simulink model "REV2_System_Model"  (R2024a)
settings: Solver=VariableStepAuto  StartTime=0.0  StopTime=10.0  RelTol=1e-3
settings Model: Creator=aniru  LastModifiedBy=aniru

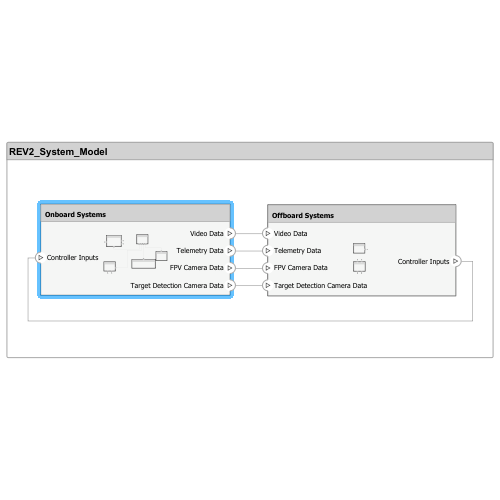
[thumbnail: Simulink's stored preview of the top-level diagram]
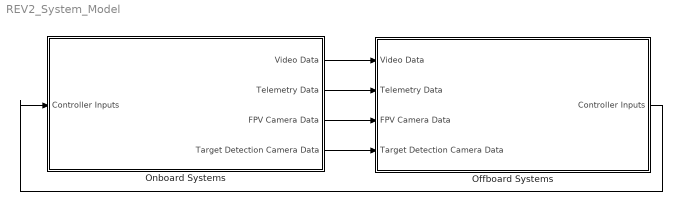
== system REV2_System_Model ==
  Offboard Systems : Subsystem
      settings: PortSchema="{\"entries\":[{\"content\":{\"headerSize\":26,\"margin\":15,\"minimumSpacing\":25,\"sides\":[{\"content\":{\"connectorIds\":[\"In2\",\"In1\",\"In4\",\"In3\"]},\"type\":\"ConnectorPlacement.EquallySpacedRectSide\",\"uuid\":\"d7d6a46a-69a6-4a79-809b-721a0c8eab4f\"},{\"content\":{\"connectorIds\":[\"Out1\"],\"side\":\"RIGHT\"},\"type\":\"ConnectorPlacement.EquallySpacedRectSide\",\"uuid\":\"fe49b777-678a-4db7-ba73-a39a909a246c\"},{\"content\":{\"side\":\"TOP\"},\"type\":\"ConnectorPlacement.EquallySpacedRectSide\",\"uuid\":\"cb797f4a-9c1e-493c-ad8d-bde4ad46238b\"}]},\"type\":\"ConnectorPlacement.EquallySpacedConnector\",\"uuid\":\"3089ea26-fd8d-45f7-b3f9-d3dc57c95d69\"}],\"packageUris\":[\"http://schema.mathworks.com/mf0/Connector/R2020b\"],\"version\":\"1.0\"}"
  Onboard Systems : Subsystem
      settings: PortSchema="{\"entries\":[{\"content\":{\"headerSize\":26,\"margin\":15,\"minimumSpacing\":25,\"sides\":[{\"content\":{\"connectorIds\":[\"In1\"]},\"type\":\"ConnectorPlacement.EquallySpacedRectSide\",\"uuid\":\"d7d6a46a-69a6-4a79-809b-721a0c8eab4f\"},{\"content\":{\"connectorIds\":[\"Out1\",\"Out2\",\"Out3\",\"Out4\"],\"side\":\"RIGHT\"},\"type\":\"ConnectorPlacement.EquallySpacedRectSide\",\"uuid\":\"fe49b777-678a-4db7-ba73-a39a909a246c\"},{\"content\":{\"side\":\"TOP\"},\"type\":\"ConnectorPlacement.EquallySpacedRectSide\",\"uuid\":\"cb797f4a-9c1e-493c-ad8d-bde4ad46238b\"}]},\"type\":\"ConnectorPlacement.EquallySpacedConnector\",\"uuid\":\"3089ea26-fd8d-45f7-b3f9-d3dc57c95d69\"}],\"packageUris\":[\"http://schema.mathworks.com/mf0/Connector/R2020b\"],\"version\":\"1.0\"}"
  wires:
  Offboard Systems/1(Controller Inputs) -> Onboard Systems/1(Controller Inputs)
  Onboard Systems/3(FPV Camera Data) -> Offboard Systems/4(FPV Camera Data)
  Onboard Systems/2(Telemetry Data) -> Offboard Systems/1(Telemetry Data)
  Onboard Systems/1(Video Data) -> Offboard Systems/2(Video Data)
  Onboard Systems/4(Target Detection Camera Data) -> Offboard Systems/3(Target Detection Camera Data)

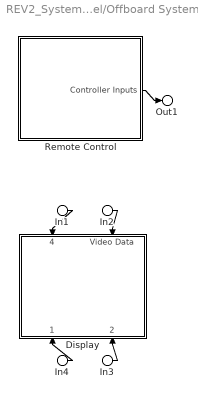
== system REV2_System_Model/Offboard Systems ==
  In1 : Inport  PortName=Telemetry Data
  In2 : Inport  Port=2  PortName=Video Data
  In3 : Inport  Port=3  PortName=Target Detection Camera Data
  In4 : Inport  Port=4  PortName=FPV Camera Data
  Display : Subsystem
      settings: PortSchema="{\"entries\":[{\"content\":{\"headerSize\":26,\"margin\":15,\"minimumSpacing\":25,\"sides\":[{\"content\":{},\"type\":\"ConnectorPlacement.EquallySpacedRectSide\",\"uuid\":\"6c101896-e527-45ce-9d84-a3c14c06145c\"},{\"content\":{\"side\":\"RIGHT\"},\"type\":\"ConnectorPlacement.EquallySpacedRectSide\",\"uuid\":\"7b64ffc1-aa7d-497e-846b-163cb9ac8cea\"},{\"content\":{\"connectorIds\":[\"In4\",\"In3\"],\"side\":\"TOP\"},\"type\":\"ConnectorPlacement.EquallySpacedRectSide\",\"uuid\":\"0b9f5c44-a735-498a-9ac1-d2acf3f6061a\"},{\"content\":{\"connectorIds\":[\"In1\",\"In2\"],\"side\":\"BOTTOM\"},\"type\":\"ConnectorPlacement.EquallySpacedRectSide\",\"uuid\":\"b98482f4-056a-41a8-96b6-ee04bf11c001\"}]},\"type\":\"ConnectorPlacement.EquallySpacedConnector\",\"uuid\":\"98444eb4-f2c3-4944-8bef-595148a64e3e\"}],\"packageUris\":[\"http://schema.mathworks.com/mf0/Connector/R2020b\"],\"version\":\"1.0\"}"
  Remote Control : Subsystem
      settings: PortSchema="{\"entries\":[{\"content\":{\"headerSize\":26,\"margin\":15,\"minimumSpacing\":25,\"sides\":[{\"content\":{},\"type\":\"ConnectorPlacement.EquallySpacedRectSide\",\"uuid\":\"6c101896-e527-45ce-9d84-a3c14c06145c\"},{\"content\":{\"connectorIds\":[\"Out1\"],\"side\":\"RIGHT\"},\"type\":\"ConnectorPlacement.EquallySpacedRectSide\",\"uuid\":\"7b64ffc1-aa7d-497e-846b-163cb9ac8cea\"},{\"content\":{\"side\":\"TOP\"},\"type\":\"ConnectorPlacement.EquallySpacedRectSide\",\"uuid\":\"0b9f5c44-a735-498a-9ac1-d2acf3f6061a\"}]},\"type\":\"ConnectorPlacement.EquallySpacedConnector\",\"uuid\":\"98444eb4-f2c3-4944-8bef-595148a64e3e\"}],\"packageUris\":[\"http://schema.mathworks.com/mf0/Connector/R2020b\"],\"version\":\"1.0\"}"
  Out1 : Outport  PortName=Controller Inputs
  wires:
  Remote Control/1(Controller Inputs) -> Out1/1
  In4/1 -> Display/1(FPV Camera Data)
  In1/1 -> Display/4(Telemetry Data)
  In3/1 -> Display/2(Target Detection Camera Data)
  In2/1 -> Display/3(Video Data)

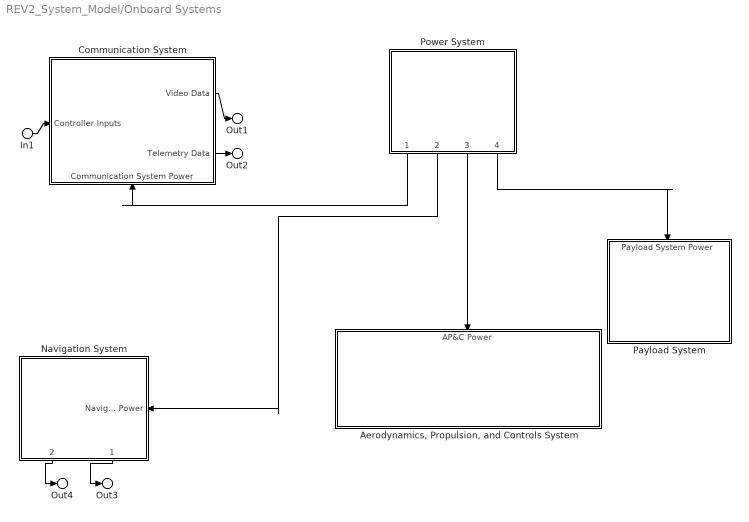
== system REV2_System_Model/Onboard Systems ==
  In1 : Inport  PortName=Controller Inputs
  "Aerodynamics, Propulsion, and Controls System" : Subsystem
      settings: PortSchema="{\"entries\":[{\"content\":{\"headerSize\":26,\"margin\":15,\"minimumSpacing\":25,\"sides\":[{\"content\":{},\"type\":\"ConnectorPlacement.EquallySpacedRectSide\",\"uuid\":\"6c101896-e527-45ce-9d84-a3c14c06145c\"},{\"content\":{\"side\":\"RIGHT\"},\"type\":\"ConnectorPlacement.EquallySpacedRectSide\",\"uuid\":\"7b64ffc1-aa7d-497e-846b-163cb9ac8cea\"},{\"content\":{\"connectorIds\":[\"In1\"],\"side\":\"TOP\"},\"type\":\"ConnectorPlacement.EquallySpacedRectSide\",\"uuid\":\"0b9f5c44-a735-498a-9ac1-d2acf3f6061a\"}]},\"type\":\"ConnectorPlacement.EquallySpacedConnector\",\"uuid\":\"98444eb4-f2c3-4944-8bef-595148a64e3e\"}],\"packageUris\":[\"http://schema.mathworks.com/mf0/Connector/R2020b\"],\"version\":\"1.0\"}"
  Communication System : Subsystem
      settings: PortSchema="{\"entries\":[{\"content\":{\"headerSize\":26,\"margin\":15,\"minimumSpacing\":25,\"sides\":[{\"content\":{\"connectorIds\":[\"In2\"]},\"type\":\"ConnectorPlacement.EquallySpacedRectSide\",\"uuid\":\"6c101896-e527-45ce-9d84-a3c14c06145c\"},{\"content\":{\"connectorIds\":[\"Out1\",\"Out2\"],\"side\":\"RIGHT\"},\"type\":\"ConnectorPlacement.EquallySpacedRectSide\",\"uuid\":\"7b64ffc1-aa7d-497e-846b-163cb9ac8cea\"},{\"content\":{\"side\":\"TOP\"},\"type\":\"ConnectorPlacement.EquallySpacedRectSide\",\"uuid\":\"0b9f5c44-a735-498a-9ac1-d2acf3f6061a\"},{\"content\":{\"connectorIds\":[\"In1\"],\"side\":\"BOTTOM\"},\"type\":\"ConnectorPlacement.EquallySpacedRectSide\",\"uuid\":\"9897a04f-e9a0-4ac0-b886-54304a1cfaaf\"}]},\"type\":\"ConnectorPlacement.EquallySpacedConnector\",\"uuid\":\"98444eb4-f2c3-4944-8bef-595148a64e3e\"}],\"packageUris\":[\"http://schema.mathworks.com/mf0/Connector/R2020b\"],\"version\":\"1.0\"}"
  Navigation System : Subsystem
      settings: PortSchema="{\"entries\":[{\"content\":{\"headerSize\":26,\"margin\":15,\"minimumSpacing\":25,\"sides\":[{\"content\":{},\"type\":\"ConnectorPlacement.EquallySpacedRectSide\",\"uuid\":\"6c101896-e527-45ce-9d84-a3c14c06145c\"},{\"content\":{\"connectorIds\":[\"In1\"],\"side\":\"RIGHT\"},\"type\":\"ConnectorPlacement.EquallySpacedRectSide\",\"uuid\":\"7b64ffc1-aa7d-497e-846b-163cb9ac8cea\"},{\"content\":{\"side\":\"TOP\"},\"type\":\"ConnectorPlacement.EquallySpacedRectSide\",\"uuid\":\"0b9f5c44-a735-498a-9ac1-d2acf3f6061a\"},{\"content\":{\"connectorIds\":[\"Out2\",\"Out1\"],\"side\":\"BOTTOM\"},\"type\":\"ConnectorPlacement.EquallySpacedRectSide\",\"uuid\":\"259bf6c7-be2f-4cef-8f2e-f10d70a04bd1\"}]},\"type\":\"ConnectorPlacement.EquallySpacedConnector\",\"uuid\":\"98444eb4-f2c3-4944-8bef-595148a64e3e\"}],\"packageUris\":[\"http://schema.mathworks.com/mf0/Connector/R2020b\"],\"version\":\"1.0\"}"
  Payload System : Subsystem
      settings: PortSchema="{\"entries\":[{\"content\":{\"headerSize\":26,\"margin\":15,\"minimumSpacing\":25,\"sides\":[{\"content\":{},\"type\":\"ConnectorPlacement.EquallySpacedRectSide\",\"uuid\":\"6c101896-e527-45ce-9d84-a3c14c06145c\"},{\"content\":{\"side\":\"RIGHT\"},\"type\":\"ConnectorPlacement.EquallySpacedRectSide\",\"uuid\":\"7b64ffc1-aa7d-497e-846b-163cb9ac8cea\"},{\"content\":{\"connectorIds\":[\"In1\"],\"side\":\"TOP\"},\"type\":\"ConnectorPlacement.EquallySpacedRectSide\",\"uuid\":\"0b9f5c44-a735-498a-9ac1-d2acf3f6061a\"}]},\"type\":\"ConnectorPlacement.EquallySpacedConnector\",\"uuid\":\"98444eb4-f2c3-4944-8bef-595148a64e3e\"}],\"packageUris\":[\"http://schema.mathworks.com/mf0/Connector/R2020b\"],\"version\":\"1.0\"}"
  Power System : Subsystem
      settings: PortSchema="{\"entries\":[{\"content\":{\"headerSize\":26,\"margin\":15,\"minimumSpacing\":25,\"sides\":[{\"content\":{},\"type\":\"ConnectorPlacement.EquallySpacedRectSide\",\"uuid\":\"6c101896-e527-45ce-9d84-a3c14c06145c\"},{\"content\":{\"side\":\"RIGHT\"},\"type\":\"ConnectorPlacement.EquallySpacedRectSide\",\"uuid\":\"7b64ffc1-aa7d-497e-846b-163cb9ac8cea\"},{\"content\":{\"side\":\"TOP\"},\"type\":\"ConnectorPlacement.EquallySpacedRectSide\",\"uuid\":\"0b9f5c44-a735-498a-9ac1-d2acf3f6061a\"},{\"content\":{\"connectorIds\":[\"Out1\",\"Out2\",\"Out3\",\"Out4\"],\"side\":\"BOTTOM\"},\"type\":\"ConnectorPlacement.EquallySpacedRectSide\",\"uuid\":\"43d6deb7-4383-40a4-bbc3-66798478452f\"}]},\"type\":\"ConnectorPlacement.EquallySpacedConnector\",\"uuid\":\"98444eb4-f2c3-4944-8bef-595148a64e3e\"}],\"packageUris\":[\"http://schema.mathworks.com/mf0/Connector/R2020b\"],\"version\":\"1.0\"}"
  Out1 : Outport  PortName=Video Data
  Out2 : Outport  Port=2  PortName=Telemetry Data
  Out3 : Outport  Port=3  PortName=FPV Camera Data
  Out4 : Outport  Port=4  PortName=Target Detection Camera Data
  wires:
  In1/1 -> Communication System/2(Controller Inputs)
  Power System/2(Navigation System Power) -> Navigation System/1(Navigation System Power)
  Navigation System/1(FPV Camera Data) -> Out3/1
  Power System/4(Payload System Power) -> Payload System/1(Payload System Power)
  Power System/3(AP&C Power) -> "Aerodynamics, Propulsion, and Controls System"/1(AP&C Power)
  Navigation System/2(Target Detection Camera Data) -> Out4/1
  Power System/1(Communication System Power) -> Communication System/1(Communication System Power)
  Communication System/1(Video Data) -> Out1/1
  Communication System/2(Telemetry Data) -> Out2/1

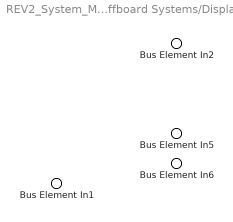
== system REV2_System_Model/Offboard Systems/Display ==
  Bus Element In6 : Inport  PortName=FPV Camera Data
  Bus Element In5 : Inport  Port=2  PortName=Target Detection Camera Data
  Bus Element In2 : Inport  Port=3  PortName=Video Data
  Bus Element In1 : Inport  Port=4  PortName=Telemetry Data

== system REV2_System_Model/Offboard Systems/Remote Control ==
  Bus Element Out1 : Outport  PortName=Controller Inputs

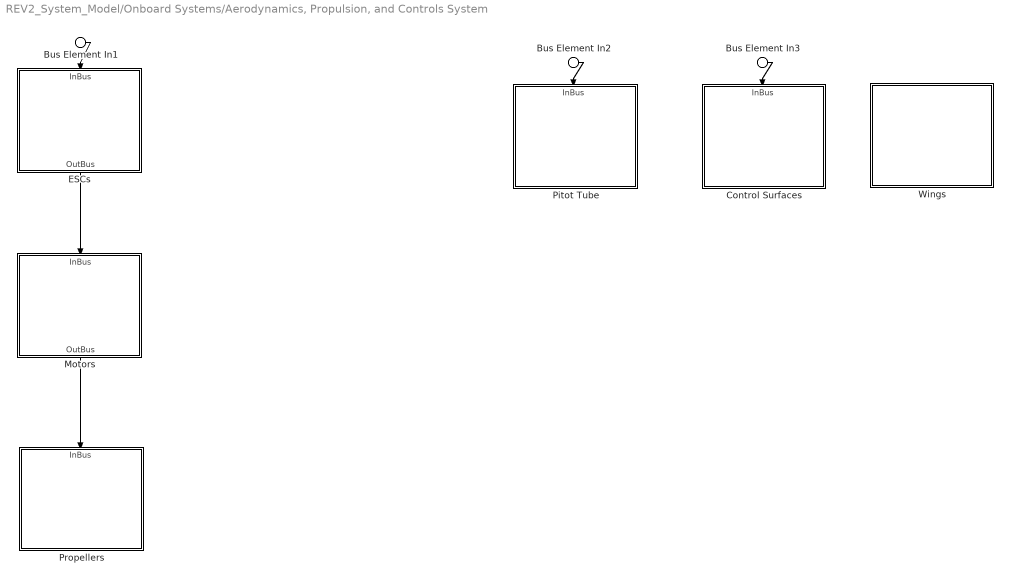
== system REV2_System_Model/Onboard Systems/Aerodynamics, Propulsion, and Controls System ==
  Bus Element In1 : Inport  PortName=AP&C Power
  Bus Element In2 : Inport  PortName=AP&C Power
  Bus Element In3 : Inport  PortName=AP&C Power
  Control Surfaces : Subsystem
      settings: PortSchema="{\"entries\":[{\"content\":{\"headerSize\":26,\"margin\":15,\"minimumSpacing\":25,\"sides\":[{\"content\":{},\"type\":\"ConnectorPlacement.EquallySpacedRectSide\",\"uuid\":\"6c101896-e527-45ce-9d84-a3c14c06145c\"},{\"content\":{\"side\":\"RIGHT\"},\"type\":\"ConnectorPlacement.EquallySpacedRectSide\",\"uuid\":\"7b64ffc1-aa7d-497e-846b-163cb9ac8cea\"},{\"content\":{\"connectorIds\":[\"In1\"],\"side\":\"TOP\"},\"type\":\"ConnectorPlacement.EquallySpacedRectSide\",\"uuid\":\"0b9f5c44-a735-498a-9ac1-d2acf3f6061a\"}]},\"type\":\"ConnectorPlacement.EquallySpacedConnector\",\"uuid\":\"98444eb4-f2c3-4944-8bef-595148a64e3e\"}],\"packageUris\":[\"http://schema.mathworks.com/mf0/Connector/R2020b\"],\"version\":\"1.0\"}"
  ESCs : Subsystem
      settings: PortSchema="{\"entries\":[{\"content\":{\"headerSize\":26,\"margin\":15,\"minimumSpacing\":25,\"sides\":[{\"content\":{},\"type\":\"ConnectorPlacement.EquallySpacedRectSide\",\"uuid\":\"6c101896-e527-45ce-9d84-a3c14c06145c\"},{\"content\":{\"side\":\"RIGHT\"},\"type\":\"ConnectorPlacement.EquallySpacedRectSide\",\"uuid\":\"7b64ffc1-aa7d-497e-846b-163cb9ac8cea\"},{\"content\":{\"connectorIds\":[\"In1\"],\"side\":\"TOP\"},\"type\":\"ConnectorPlacement.EquallySpacedRectSide\",\"uuid\":\"0b9f5c44-a735-498a-9ac1-d2acf3f6061a\"},{\"content\":{\"connectorIds\":[\"Out1\"],\"side\":\"BOTTOM\"},\"type\":\"ConnectorPlacement.EquallySpacedRectSide\",\"uuid\":\"e6155134-ab54-484f-884a-95cc513b47d0\"}]},\"type\":\"ConnectorPlacement.EquallySpacedConnector\",\"uuid\":\"98444eb4-f2c3-4944-8bef-595148a64e3e\"}],\"packageUris\":[\"http://schema.mathworks.com/mf0/Connector/R2020b\"],\"version\":\"1.0\"}"
  Motors : Subsystem
      settings: PortSchema="{\"entries\":[{\"content\":{\"headerSize\":26,\"margin\":15,\"minimumSpacing\":25,\"sides\":[{\"content\":{},\"type\":\"ConnectorPlacement.EquallySpacedRectSide\",\"uuid\":\"6c101896-e527-45ce-9d84-a3c14c06145c\"},{\"content\":{\"side\":\"RIGHT\"},\"type\":\"ConnectorPlacement.EquallySpacedRectSide\",\"uuid\":\"7b64ffc1-aa7d-497e-846b-163cb9ac8cea\"},{\"content\":{\"connectorIds\":[\"In1\"],\"side\":\"TOP\"},\"type\":\"ConnectorPlacement.EquallySpacedRectSide\",\"uuid\":\"0b9f5c44-a735-498a-9ac1-d2acf3f6061a\"},{\"content\":{\"connectorIds\":[\"Out1\"],\"side\":\"BOTTOM\"},\"type\":\"ConnectorPlacement.EquallySpacedRectSide\",\"uuid\":\"bcf1fd8b-32d5-427a-a7f4-b07a8b3a016f\"}]},\"type\":\"ConnectorPlacement.EquallySpacedConnector\",\"uuid\":\"98444eb4-f2c3-4944-8bef-595148a64e3e\"}],\"packageUris\":[\"http://schema.mathworks.com/mf0/Connector/R2020b\"],\"version\":\"1.0\"}"
  Pitot Tube : Subsystem
      settings: PortSchema="{\"entries\":[{\"content\":{\"headerSize\":26,\"margin\":15,\"minimumSpacing\":25,\"sides\":[{\"content\":{},\"type\":\"ConnectorPlacement.EquallySpacedRectSide\",\"uuid\":\"6c101896-e527-45ce-9d84-a3c14c06145c\"},{\"content\":{\"side\":\"RIGHT\"},\"type\":\"ConnectorPlacement.EquallySpacedRectSide\",\"uuid\":\"7b64ffc1-aa7d-497e-846b-163cb9ac8cea\"},{\"content\":{\"connectorIds\":[\"In1\"],\"side\":\"TOP\"},\"type\":\"ConnectorPlacement.EquallySpacedRectSide\",\"uuid\":\"0b9f5c44-a735-498a-9ac1-d2acf3f6061a\"}]},\"type\":\"ConnectorPlacement.EquallySpacedConnector\",\"uuid\":\"98444eb4-f2c3-4944-8bef-595148a64e3e\"}],\"packageUris\":[\"http://schema.mathworks.com/mf0/Connector/R2020b\"],\"version\":\"1.0\"}"
  Propellers : Subsystem
      settings: PortSchema="{\"entries\":[{\"content\":{\"headerSize\":26,\"margin\":15,\"minimumSpacing\":25,\"sides\":[{\"content\":{},\"type\":\"ConnectorPlacement.EquallySpacedRectSide\",\"uuid\":\"6c101896-e527-45ce-9d84-a3c14c06145c\"},{\"content\":{\"side\":\"RIGHT\"},\"type\":\"ConnectorPlacement.EquallySpacedRectSide\",\"uuid\":\"7b64ffc1-aa7d-497e-846b-163cb9ac8cea\"},{\"content\":{\"connectorIds\":[\"In1\"],\"side\":\"TOP\"},\"type\":\"ConnectorPlacement.EquallySpacedRectSide\",\"uuid\":\"0b9f5c44-a735-498a-9ac1-d2acf3f6061a\"}]},\"type\":\"ConnectorPlacement.EquallySpacedConnector\",\"uuid\":\"98444eb4-f2c3-4944-8bef-595148a64e3e\"}],\"packageUris\":[\"http://schema.mathworks.com/mf0/Connector/R2020b\"],\"version\":\"1.0\"}"
  Wings : Subsystem
      settings: PortSchema="{\"entries\":[{\"content\":{\"headerSize\":26,\"margin\":15,\"minimumSpacing\":25,\"sides\":[{\"content\":{},\"type\":\"ConnectorPlacement.EquallySpacedRectSide\",\"uuid\":\"6c101896-e527-45ce-9d84-a3c14c06145c\"},{\"content\":{\"side\":\"RIGHT\"},\"type\":\"ConnectorPlacement.EquallySpacedRectSide\",\"uuid\":\"7b64ffc1-aa7d-497e-846b-163cb9ac8cea\"},{\"content\":{\"side\":\"TOP\"},\"type\":\"ConnectorPlacement.EquallySpacedRectSide\",\"uuid\":\"0b9f5c44-a735-498a-9ac1-d2acf3f6061a\"}]},\"type\":\"ConnectorPlacement.EquallySpacedConnector\",\"uuid\":\"98444eb4-f2c3-4944-8bef-595148a64e3e\"}],\"packageUris\":[\"http://schema.mathworks.com/mf0/Connector/R2020b\"],\"version\":\"1.0\"}"
  wires:
  Bus Element In1/1 -> ESCs/1(InBus)
  ESCs/1(OutBus) -> Motors/1(InBus)
  Motors/1(OutBus) -> Propellers/1(InBus)
  Bus Element In2/1 -> Pitot Tube/1(InBus)
  Bus Element In3/1 -> Control Surfaces/1(InBus)

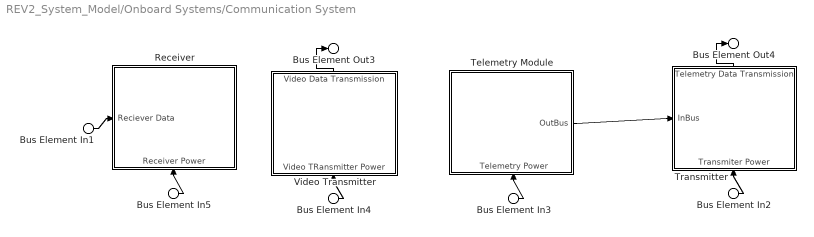
== system REV2_System_Model/Onboard Systems/Communication System ==
  Bus Element In{2..5} (4 alike) : Inport  PortName=Communication System Power
  Bus Element In1 : Inport  Port=2  PortName=Controller Inputs
  Receiver : Subsystem
      settings: PortSchema="{\"entries\":[{\"content\":{\"headerSize\":26,\"margin\":15,\"minimumSpacing\":25,\"sides\":[{\"content\":{\"connectorIds\":[\"In2\"]},\"type\":\"ConnectorPlacement.EquallySpacedRectSide\",\"uuid\":\"6c101896-e527-45ce-9d84-a3c14c06145c\"},{\"content\":{\"side\":\"RIGHT\"},\"type\":\"ConnectorPlacement.EquallySpacedRectSide\",\"uuid\":\"7b64ffc1-aa7d-497e-846b-163cb9ac8cea\"},{\"content\":{\"side\":\"TOP\"},\"type\":\"ConnectorPlacement.EquallySpacedRectSide\",\"uuid\":\"0b9f5c44-a735-498a-9ac1-d2acf3f6061a\"},{\"content\":{\"connectorIds\":[\"In1\"],\"side\":\"BOTTOM\"},\"type\":\"ConnectorPlacement.EquallySpacedRectSide\",\"uuid\":\"225c5263-079d-4e6f-92ca-e038b253b7aa\"}]},\"type\":\"ConnectorPlacement.EquallySpacedConnector\",\"uuid\":\"98444eb4-f2c3-4944-8bef-595148a64e3e\"}],\"packageUris\":[\"http://schema.mathworks.com/mf0/Connector/R2020b\"],\"version\":\"1.0\"}"
  Telemetry Module : Subsystem
      settings: PortSchema="{\"entries\":[{\"content\":{\"headerSize\":26,\"margin\":15,\"minimumSpacing\":25,\"sides\":[{\"content\":{},\"type\":\"ConnectorPlacement.EquallySpacedRectSide\",\"uuid\":\"6c101896-e527-45ce-9d84-a3c14c06145c\"},{\"content\":{\"connectorIds\":[\"Out1\"],\"side\":\"RIGHT\"},\"type\":\"ConnectorPlacement.EquallySpacedRectSide\",\"uuid\":\"7b64ffc1-aa7d-497e-846b-163cb9ac8cea\"},{\"content\":{\"side\":\"TOP\"},\"type\":\"ConnectorPlacement.EquallySpacedRectSide\",\"uuid\":\"0b9f5c44-a735-498a-9ac1-d2acf3f6061a\"},{\"content\":{\"connectorIds\":[\"In1\"],\"side\":\"BOTTOM\"},\"type\":\"ConnectorPlacement.EquallySpacedRectSide\",\"uuid\":\"eabf0b1b-1ec2-48b3-a848-f629f6867108\"}]},\"type\":\"ConnectorPlacement.EquallySpacedConnector\",\"uuid\":\"98444eb4-f2c3-4944-8bef-595148a64e3e\"}],\"packageUris\":[\"http://schema.mathworks.com/mf0/Connector/R2020b\"],\"version\":\"1.0\"}"
  Transmitter : Subsystem
      settings: PortSchema="{\"entries\":[{\"content\":{\"headerSize\":26,\"margin\":15,\"minimumSpacing\":25,\"sides\":[{\"content\":{\"connectorIds\":[\"In2\"]},\"type\":\"ConnectorPlacement.EquallySpacedRectSide\",\"uuid\":\"6c101896-e527-45ce-9d84-a3c14c06145c\"},{\"content\":{\"side\":\"RIGHT\"},\"type\":\"ConnectorPlacement.EquallySpacedRectSide\",\"uuid\":\"7b64ffc1-aa7d-497e-846b-163cb9ac8cea\"},{\"content\":{\"connectorIds\":[\"Out1\"],\"side\":\"TOP\"},\"type\":\"ConnectorPlacement.EquallySpacedRectSide\",\"uuid\":\"0b9f5c44-a735-498a-9ac1-d2acf3f6061a\"},{\"content\":{\"connectorIds\":[\"In1\"],\"side\":\"BOTTOM\"},\"type\":\"ConnectorPlacement.EquallySpacedRectSide\",\"uuid\":\"a557d3ac-4447-49b7-a233-853cfdf461ae\"}]},\"type\":\"ConnectorPlacement.EquallySpacedConnector\",\"uuid\":\"98444eb4-f2c3-4944-8bef-595148a64e3e\"}],\"packageUris\":[\"http://schema.mathworks.com/mf0/Connector/R2020b\"],\"version\":\"1.0\"}"
  Video Transmitter : Subsystem
      settings: PortSchema="{\"entries\":[{\"content\":{\"headerSize\":26,\"margin\":15,\"minimumSpacing\":25,\"sides\":[{\"content\":{},\"type\":\"ConnectorPlacement.EquallySpacedRectSide\",\"uuid\":\"6c101896-e527-45ce-9d84-a3c14c06145c\"},{\"content\":{\"side\":\"RIGHT\"},\"type\":\"ConnectorPlacement.EquallySpacedRectSide\",\"uuid\":\"7b64ffc1-aa7d-497e-846b-163cb9ac8cea\"},{\"content\":{\"connectorIds\":[\"Out1\"],\"side\":\"TOP\"},\"type\":\"ConnectorPlacement.EquallySpacedRectSide\",\"uuid\":\"0b9f5c44-a735-498a-9ac1-d2acf3f6061a\"},{\"content\":{\"connectorIds\":[\"In1\"],\"side\":\"BOTTOM\"},\"type\":\"ConnectorPlacement.EquallySpacedRectSide\",\"uuid\":\"9b6e493b-9887-4837-832b-8322a949f735\"}]},\"type\":\"ConnectorPlacement.EquallySpacedConnector\",\"uuid\":\"98444eb4-f2c3-4944-8bef-595148a64e3e\"}],\"packageUris\":[\"http://schema.mathworks.com/mf0/Connector/R2020b\"],\"version\":\"1.0\"}"
  Bus Element Out3 : Outport  PortName=Video Data
  Bus Element Out4 : Outport  Port=2  PortName=Telemetry Data
  wires:
  Telemetry Module/1(OutBus) -> Transmitter/2(InBus)
  Transmitter/1(Telemetry Data Transmission) -> Bus Element Out4/1
  Video Transmitter/1(Video Data Transmission) -> Bus Element Out3/1
  Bus Element In2/1 -> Transmitter/1(Transmiter Power)
  Bus Element In3/1 -> Telemetry Module/1(Telemetry Power)
  Bus Element In4/1 -> Video Transmitter/1(Video TRansmitter Power)
  Bus Element In5/1 -> Receiver/1(Receiver Power)
  Bus Element In1/1 -> Receiver/2(Reciever Data)

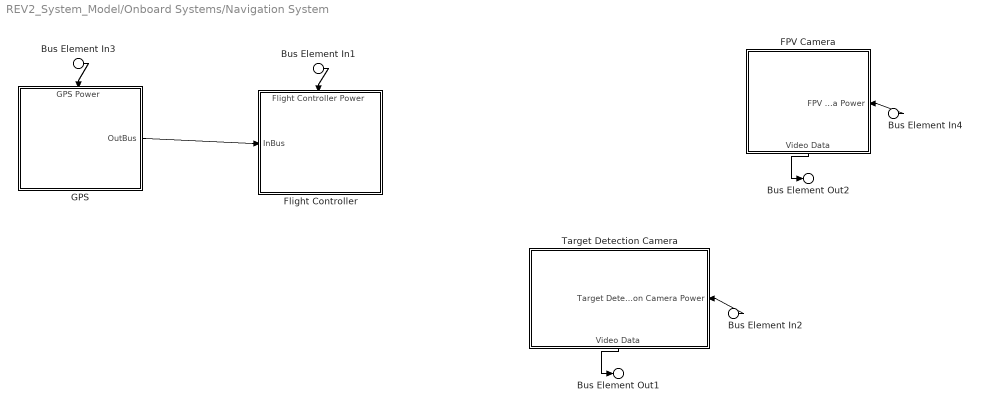
== system REV2_System_Model/Onboard Systems/Navigation System ==
  Bus Element In{1..4} (4 alike) : Inport  PortName=Navigation System Power
  FPV Camera : Subsystem
      settings: PortSchema="{\"entries\":[{\"content\":{\"headerSize\":26,\"margin\":15,\"minimumSpacing\":25,\"sides\":[{\"content\":{},\"type\":\"ConnectorPlacement.EquallySpacedRectSide\",\"uuid\":\"6c101896-e527-45ce-9d84-a3c14c06145c\"},{\"content\":{\"connectorIds\":[\"In1\"],\"side\":\"RIGHT\"},\"type\":\"ConnectorPlacement.EquallySpacedRectSide\",\"uuid\":\"7b64ffc1-aa7d-497e-846b-163cb9ac8cea\"},{\"content\":{\"side\":\"TOP\"},\"type\":\"ConnectorPlacement.EquallySpacedRectSide\",\"uuid\":\"0b9f5c44-a735-498a-9ac1-d2acf3f6061a\"},{\"content\":{\"connectorIds\":[\"Out1\"],\"side\":\"BOTTOM\"},\"type\":\"ConnectorPlacement.EquallySpacedRectSide\",\"uuid\":\"a58eef8c-833a-469f-9edc-d38f32c82231\"}]},\"type\":\"ConnectorPlacement.EquallySpacedConnector\",\"uuid\":\"98444eb4-f2c3-4944-8bef-595148a64e3e\"}],\"packageUris\":[\"http://schema.mathworks.com/mf0/Connector/R2020b\"],\"version\":\"1.0\"}"
  Flight Controller : Subsystem
      settings: PortSchema="{\"entries\":[{\"content\":{\"headerSize\":26,\"margin\":15,\"minimumSpacing\":25,\"sides\":[{\"content\":{\"connectorIds\":[\"In2\"]},\"type\":\"ConnectorPlacement.EquallySpacedRectSide\",\"uuid\":\"6c101896-e527-45ce-9d84-a3c14c06145c\"},{\"content\":{\"side\":\"RIGHT\"},\"type\":\"ConnectorPlacement.EquallySpacedRectSide\",\"uuid\":\"7b64ffc1-aa7d-497e-846b-163cb9ac8cea\"},{\"content\":{\"connectorIds\":[\"In1\"],\"side\":\"TOP\"},\"type\":\"ConnectorPlacement.EquallySpacedRectSide\",\"uuid\":\"0b9f5c44-a735-498a-9ac1-d2acf3f6061a\"}]},\"type\":\"ConnectorPlacement.EquallySpacedConnector\",\"uuid\":\"98444eb4-f2c3-4944-8bef-595148a64e3e\"}],\"packageUris\":[\"http://schema.mathworks.com/mf0/Connector/R2020b\"],\"version\":\"1.0\"}"
  GPS : Subsystem
      settings: PortSchema="{\"entries\":[{\"content\":{\"headerSize\":26,\"margin\":15,\"minimumSpacing\":25,\"sides\":[{\"content\":{},\"type\":\"ConnectorPlacement.EquallySpacedRectSide\",\"uuid\":\"6c101896-e527-45ce-9d84-a3c14c06145c\"},{\"content\":{\"connectorIds\":[\"Out1\"],\"side\":\"RIGHT\"},\"type\":\"ConnectorPlacement.EquallySpacedRectSide\",\"uuid\":\"7b64ffc1-aa7d-497e-846b-163cb9ac8cea\"},{\"content\":{\"connectorIds\":[\"In1\"],\"side\":\"TOP\"},\"type\":\"ConnectorPlacement.EquallySpacedRectSide\",\"uuid\":\"0b9f5c44-a735-498a-9ac1-d2acf3f6061a\"}]},\"type\":\"ConnectorPlacement.EquallySpacedConnector\",\"uuid\":\"98444eb4-f2c3-4944-8bef-595148a64e3e\"}],\"packageUris\":[\"http://schema.mathworks.com/mf0/Connector/R2020b\"],\"version\":\"1.0\"}"
  Target Detection Camera : Subsystem
      settings: PortSchema="{\"entries\":[{\"content\":{\"headerSize\":26,\"margin\":15,\"minimumSpacing\":25,\"sides\":[{\"content\":{},\"type\":\"ConnectorPlacement.EquallySpacedRectSide\",\"uuid\":\"6c101896-e527-45ce-9d84-a3c14c06145c\"},{\"content\":{\"connectorIds\":[\"In1\"],\"side\":\"RIGHT\"},\"type\":\"ConnectorPlacement.EquallySpacedRectSide\",\"uuid\":\"7b64ffc1-aa7d-497e-846b-163cb9ac8cea\"},{\"content\":{\"side\":\"TOP\"},\"type\":\"ConnectorPlacement.EquallySpacedRectSide\",\"uuid\":\"0b9f5c44-a735-498a-9ac1-d2acf3f6061a\"},{\"content\":{\"connectorIds\":[\"Out1\"],\"side\":\"BOTTOM\"},\"type\":\"ConnectorPlacement.EquallySpacedRectSide\",\"uuid\":\"94a18fa8-c1d9-4804-bbf1-fc9d2a932311\"}]},\"type\":\"ConnectorPlacement.EquallySpacedConnector\",\"uuid\":\"98444eb4-f2c3-4944-8bef-595148a64e3e\"}],\"packageUris\":[\"http://schema.mathworks.com/mf0/Connector/R2020b\"],\"version\":\"1.0\"}"
  Bus Element Out2 : Outport  PortName=FPV Camera Data
  Bus Element Out1 : Outport  Port=2  PortName=Target Detection Camera Data
  wires:
  GPS/1(OutBus) -> Flight Controller/2(InBus)
  Bus Element In1/1 -> Flight Controller/1(Flight Controller Power)
  Target Detection Camera/1(Video Data) -> Bus Element Out1/1
  FPV Camera/1(Video Data) -> Bus Element Out2/1
  Bus Element In2/1 -> Target Detection Camera/1(Target Detection Camera Power)
  Bus Element In3/1 -> GPS/1(GPS Power)
  Bus Element In4/1 -> FPV Camera/1(FPV Camera Power)

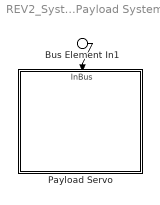
== system REV2_System_Model/Onboard Systems/Payload System ==
  Bus Element In1 : Inport  PortName=Payload System Power
  Payload Servo : Subsystem
      settings: PortSchema="{\"entries\":[{\"content\":{\"headerSize\":26,\"margin\":15,\"minimumSpacing\":25,\"sides\":[{\"content\":{},\"type\":\"ConnectorPlacement.EquallySpacedRectSide\",\"uuid\":\"6c101896-e527-45ce-9d84-a3c14c06145c\"},{\"content\":{\"side\":\"RIGHT\"},\"type\":\"ConnectorPlacement.EquallySpacedRectSide\",\"uuid\":\"7b64ffc1-aa7d-497e-846b-163cb9ac8cea\"},{\"content\":{\"connectorIds\":[\"In1\"],\"side\":\"TOP\"},\"type\":\"ConnectorPlacement.EquallySpacedRectSide\",\"uuid\":\"0b9f5c44-a735-498a-9ac1-d2acf3f6061a\"}]},\"type\":\"ConnectorPlacement.EquallySpacedConnector\",\"uuid\":\"98444eb4-f2c3-4944-8bef-595148a64e3e\"}],\"packageUris\":[\"http://schema.mathworks.com/mf0/Connector/R2020b\"],\"version\":\"1.0\"}"
  wires:
  Bus Element In1/1 -> Payload Servo/1(InBus)

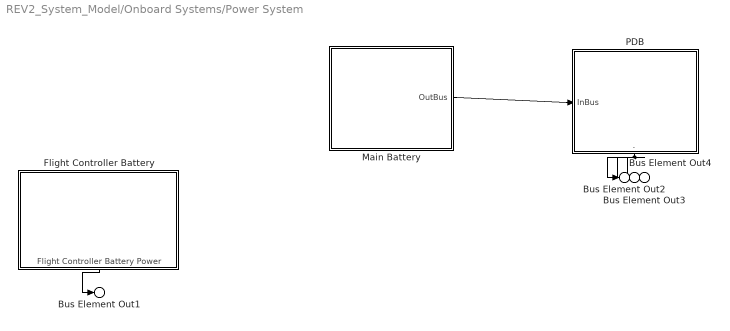
== system REV2_System_Model/Onboard Systems/Power System ==
  Flight Controller Battery : Subsystem
      settings: PortSchema="{\"entries\":[{\"content\":{\"headerSize\":26,\"margin\":15,\"minimumSpacing\":25,\"sides\":[{\"content\":{},\"type\":\"ConnectorPlacement.EquallySpacedRectSide\",\"uuid\":\"6c101896-e527-45ce-9d84-a3c14c06145c\"},{\"content\":{\"side\":\"RIGHT\"},\"type\":\"ConnectorPlacement.EquallySpacedRectSide\",\"uuid\":\"7b64ffc1-aa7d-497e-846b-163cb9ac8cea\"},{\"content\":{\"side\":\"TOP\"},\"type\":\"ConnectorPlacement.EquallySpacedRectSide\",\"uuid\":\"0b9f5c44-a735-498a-9ac1-d2acf3f6061a\"},{\"content\":{\"connectorIds\":[\"Out1\"],\"side\":\"BOTTOM\"},\"type\":\"ConnectorPlacement.EquallySpacedRectSide\",\"uuid\":\"50f8d553-bb5a-4ab8-ba1c-5e05ca9d6fce\"}]},\"type\":\"ConnectorPlacement.EquallySpacedConnector\",\"uuid\":\"98444eb4-f2c3-4944-8bef-595148a64e3e\"}],\"packageUris\":[\"http://schema.mathworks.com/mf0/Connector/R2020b\"],\"version\":\"1.0\"}"
  Main Battery : Subsystem
      settings: PortSchema="{\"entries\":[{\"content\":{\"headerSize\":26,\"margin\":15,\"minimumSpacing\":25,\"sides\":[{\"content\":{},\"type\":\"ConnectorPlacement.EquallySpacedRectSide\",\"uuid\":\"6c101896-e527-45ce-9d84-a3c14c06145c\"},{\"content\":{\"connectorIds\":[\"Out1\"],\"side\":\"RIGHT\"},\"type\":\"ConnectorPlacement.EquallySpacedRectSide\",\"uuid\":\"7b64ffc1-aa7d-497e-846b-163cb9ac8cea\"},{\"content\":{\"side\":\"TOP\"},\"type\":\"ConnectorPlacement.EquallySpacedRectSide\",\"uuid\":\"0b9f5c44-a735-498a-9ac1-d2acf3f6061a\"}]},\"type\":\"ConnectorPlacement.EquallySpacedConnector\",\"uuid\":\"98444eb4-f2c3-4944-8bef-595148a64e3e\"}],\"packageUris\":[\"http://schema.mathworks.com/mf0/Connector/R2020b\"],\"version\":\"1.0\"}"
  PDB : Subsystem
      settings: PortSchema="{\"entries\":[{\"content\":{\"headerSize\":26,\"margin\":15,\"minimumSpacing\":25,\"sides\":[{\"content\":{\"connectorIds\":[\"In1\"]},\"type\":\"ConnectorPlacement.EquallySpacedRectSide\",\"uuid\":\"6c101896-e527-45ce-9d84-a3c14c06145c\"},{\"content\":{\"side\":\"RIGHT\"},\"type\":\"ConnectorPlacement.EquallySpacedRectSide\",\"uuid\":\"7b64ffc1-aa7d-497e-846b-163cb9ac8cea\"},{\"content\":{\"side\":\"TOP\"},\"type\":\"ConnectorPlacement.EquallySpacedRectSide\",\"uuid\":\"0b9f5c44-a735-498a-9ac1-d2acf3f6061a\"},{\"content\":{\"connectorIds\":[\"Out1\"],\"side\":\"BOTTOM\"},\"type\":\"ConnectorPlacement.EquallySpacedRectSide\",\"uuid\":\"5de3aea3-c002-4c2c-8cb8-8c0a5d3edab6\"}]},\"type\":\"ConnectorPlacement.EquallySpacedConnector\",\"uuid\":\"98444eb4-f2c3-4944-8bef-595148a64e3e\"}],\"packageUris\":[\"http://schema.mathworks.com/mf0/Connector/R2020b\"],\"version\":\"1.0\"}"
  Bus Element Out4 : Outport  PortName=Communication System Power
  Bus Element Out1 : Outport  Port=2  PortName=Navigation System Power
  Bus Element Out2 : Outport  Port=3  PortName=AP&C Power
  Bus Element Out3 : Outport  Port=4  PortName=Payload System Power
  wires:
  Main Battery/1(OutBus) -> PDB/1(InBus)
  Flight Controller Battery/1(Flight Controller Battery Power) -> Bus Element Out1/1
  PDB/1(.) -> Bus Element Out4/1, Bus Element Out3/1, Bus Element Out2/1

== system REV2_System_Model/Onboard Systems/Aerodynamics, Propulsion, and Controls System/Control Surfaces ==
  Bus Element In1 : Inport  PortName=InBus

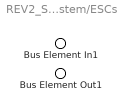
== system REV2_System_Model/Onboard Systems/Aerodynamics, Propulsion, and Controls System/ESCs ==
  Bus Element In1 : Inport  PortName=InBus
  Bus Element Out1 : Outport  PortName=OutBus

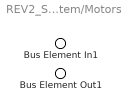
== system REV2_System_Model/Onboard Systems/Aerodynamics, Propulsion, and Controls System/Motors ==
  Bus Element In1 : Inport  PortName=InBus
  Bus Element Out1 : Outport  PortName=OutBus

== system REV2_System_Model/Onboard Systems/Aerodynamics, Propulsion, and Controls System/Pitot Tube ==
  Bus Element In1 : Inport  PortName=InBus

== system REV2_System_Model/Onboard Systems/Aerodynamics, Propulsion, and Controls System/Propellers ==
  Bus Element In1 : Inport  PortName=InBus

== system REV2_System_Model/Onboard Systems/Aerodynamics, Propulsion, and Controls System/Wings ==

== system REV2_System_Model/Onboard Systems/Communication System/Receiver ==
  Bus Element In2 : Inport  PortName=Receiver Power
  Bus Element In1 : Inport  Port=2  PortName=Reciever Data

== system REV2_System_Model/Onboard Systems/Communication System/Telemetry Module ==
  Bus Element In1 : Inport  PortName=Telemetry Power
  Bus Element Out1 : Outport  PortName=OutBus

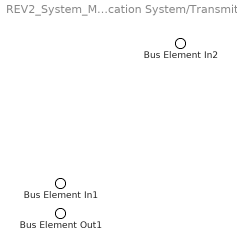
== system REV2_System_Model/Onboard Systems/Communication System/Transmitter ==
  Bus Element In2 : Inport  PortName=Transmiter Power
  Bus Element In1 : Inport  Port=2  PortName=InBus
  Bus Element Out1 : Outport  PortName=Telemetry Data Transmission

== system REV2_System_Model/Onboard Systems/Communication System/Video Transmitter ==
  Bus Element In1 : Inport  PortName=Video TRansmitter Power
  Bus Element Out1 : Outport  PortName=Video Data Transmission

== system REV2_System_Model/Onboard Systems/Navigation System/FPV Camera ==
  Bus Element In1 : Inport  PortName=FPV Camera Power
  Bus Element Out1 : Outport  PortName=Video Data

== system REV2_System_Model/Onboard Systems/Navigation System/Flight Controller ==
  Bus Element In2 : Inport  PortName=Flight Controller Power
  Bus Element In1 : Inport  Port=2  PortName=InBus

== system REV2_System_Model/Onboard Systems/Navigation System/GPS ==
  Bus Element In1 : Inport  PortName=GPS Power
  Bus Element Out1 : Outport  PortName=OutBus

== system REV2_System_Model/Onboard Systems/Navigation System/Target Detection Camera ==
  Bus Element In1 : Inport  PortName=Target Detection Camera Power
  Bus Element Out1 : Outport  PortName=Video Data

== system REV2_System_Model/Onboard Systems/Payload System/Payload Servo ==
  Bus Element In1 : Inport  PortName=InBus

== system REV2_System_Model/Onboard Systems/Power System/Flight Controller Battery ==
  Bus Element Out1 : Outport  PortName=Flight Controller Battery Power

== system REV2_System_Model/Onboard Systems/Power System/Main Battery ==
  Bus Element Out1 : Outport  PortName=OutBus

== system REV2_System_Model/Onboard Systems/Power System/PDB ==
  Bus Element In1 : Inport  PortName=InBus
  Bus Element Out1 : Outport  PortName=.
